simulink library "halin"  (R2021b)
settings: Solver=VariableStepAuto  StartTime=0.0  StopTime=10.0  RelTol=1e-3
undefined symbols (not defined in the file): KHAL_CAN1ABM1E2E_flg, KHAL_CAN1EPB1E2E_flg, KHAL_CAN1EPS1E2E_flg, KHAL_CAN1ESC1E2E_flg, KHAL_CAN1ESC5E2E_flg, KHAL_CAN3BMS1E2E_flg, KHAL_CAN3BMS6E2E_flg, KHAL_CAN3CCU1E2E_flg, KHAL_CAN3CCU2E2E_flg, KHAL_CAN3MCUNF1E2E_flg, KHAL_CAN3MCUNR1E2E_flg, KHAL_CAN3Shifter1E2E_flg, KHAL_CAN3Shifter2E2E_flg, KHAL_CAN6FCM2E2E_flg, KHAL_CAN6FCM4E2E_flg, TRUE
libraries: simulink x645, FVT_lib x212, hcu_lib x59
(part 23 of 23)

== system halin/HAL_IN/CAN6/FCM1/ForceLowBeam ==
  ForceLowBeam : Inport
  UnitConverter : DataTypeConversion  OutDataTypeStr=uint8
  VHAL_ForceLowBeam_enum : Outport
  wires:
  UnitConverter/1 -> VHAL_ForceLowBeam_enum/1
  ForceLowBeam/1 -> UnitConverter/1

== system halin/HAL_IN/CAN6/FCM1/HazardWarningReq ==
  HazardWarningReq : Inport
  UnitConverter : DataTypeConversion  OutDataTypeStr=uint8
  VHAL_HazardWarningReq_flg : Outport
  wires:
  UnitConverter/1 -> VHAL_HazardWarningReq_flg/1
  HazardWarningReq/1 -> UnitConverter/1

== system halin/HAL_IN/CAN6/FCM1/ISAWarningMsg ==
  ISA_WarningMsg : Inport
  UnitConverter : DataTypeConversion  OutDataTypeStr=uint8
  VHAL_ISAWarningMsg_enum : Outport
  wires:
  UnitConverter/1 -> VHAL_ISAWarningMsg_enum/1
  ISA_WarningMsg/1 -> UnitConverter/1

== system halin/HAL_IN/CAN6/FCM1/LKAHODDisplayWarning ==
  LKA_HOD_Display_Warning : Inport
  UnitConverter : DataTypeConversion  OutDataTypeStr=uint8
  VHAL_LKAHODDisplayWarning_flg : Outport
  wires:
  UnitConverter/1 -> VHAL_LKAHODDisplayWarning_flg/1
  LKA_HOD_Display_Warning/1 -> UnitConverter/1

== system halin/HAL_IN/CAN6/FCM1/LKAHODSoundWarning ==
  LKA_HOD_Sound_Warning : Inport
  UnitConverter : DataTypeConversion  OutDataTypeStr=uint8
  VHAL_LKAHODSoundWarning_flg : Outport
  wires:
  UnitConverter/1 -> VHAL_LKAHODSoundWarning_flg/1
  LKA_HOD_Sound_Warning/1 -> UnitConverter/1

== system halin/HAL_IN/CAN6/FCM1/LVDAACCStatusInformation ==
  LVDA_ACCStatusInformation : Inport
  UnitConverter : DataTypeConversion  OutDataTypeStr=uint8
  VHAL_LVDAACCStatusInformation_flg : Outport
  wires:
  UnitConverter/1 -> VHAL_LVDAACCStatusInformation_flg/1
  LVDA_ACCStatusInformation/1 -> UnitConverter/1

== system halin/HAL_IN/CAN6/FCM1/LVDADisabled ==
  LVDA_Disabled : Inport
  UnitConverter : DataTypeConversion  OutDataTypeStr=uint8
  VHAL_LVDADisabled_flg : Outport
  wires:
  UnitConverter/1 -> VHAL_LVDADisabled_flg/1
  LVDA_Disabled/1 -> UnitConverter/1

== system halin/HAL_IN/CAN6/FCM1/LVDAFailinfo ==
  LVDA_Failinfo : Inport
  UnitConverter : DataTypeConversion  OutDataTypeStr=uint8
  VHAL_LVDAFailinfo_flg : Outport
  wires:
  UnitConverter/1 -> VHAL_LVDAFailinfo_flg/1
  LVDA_Failinfo/1 -> UnitConverter/1

== system halin/HAL_IN/CAN6/FCM1/LVDAMuteSta ==
  LVDA_Mute_Sta : Inport
  UnitConverter : DataTypeConversion  OutDataTypeStr=uint8
  VHAL_LVDAMuteSta_enum : Outport
  wires:
  UnitConverter/1 -> VHAL_LVDAMuteSta_enum/1
  LVDA_Mute_Sta/1 -> UnitConverter/1

== system halin/HAL_IN/CAN6/FCM1/LVDAWarning ==
  LVDA_Warning : Inport
  UnitConverter : DataTypeConversion  OutDataTypeStr=uint8
  VHAL_LVDAWarning_flg : Outport
  wires:
  UnitConverter/1 -> VHAL_LVDAWarning_flg/1
  LVDA_Warning/1 -> UnitConverter/1

== system halin/HAL_IN/CAN6/FCM1/LeftTurnLightReq ==
  LeftTurnLightReq : Inport
  UnitConverter : DataTypeConversion  OutDataTypeStr=uint8
  VHAL_LeftTurnLightReq_flg : Outport
  wires:
  UnitConverter/1 -> VHAL_LeftTurnLightReq_flg/1
  LeftTurnLightReq/1 -> UnitConverter/1

== system halin/HAL_IN/CAN6/FCM1/RightTurnLightReq ==
  RightTurnLightReq : Inport
  UnitConverter : DataTypeConversion  OutDataTypeStr=uint8
  VHAL_RightTurnLightReq_flg : Outport
  wires:
  UnitConverter/1 -> VHAL_RightTurnLightReq_flg/1
  RightTurnLightReq/1 -> UnitConverter/1

== system halin/HAL_IN/CAN6/FCM1/TargetType ==
  Target_Type : Inport
  UnitConverter : DataTypeConversion  OutDataTypeStr=uint16
  VHAL_TargetType_enum : Outport
  wires:
  UnitConverter/1 -> VHAL_TargetType_enum/1
  Target_Type/1 -> UnitConverter/1

== system halin/HAL_IN/CAN6/FCM1/TimeGapLevel ==
  TimeGapLevel : Inport
  UnitConverter : DataTypeConversion  OutDataTypeStr=uint8
  VHAL_TimeGapLevel_enum : Outport
  wires:
  UnitConverter/1 -> VHAL_TimeGapLevel_enum/1
  TimeGapLevel/1 -> UnitConverter/1

== system halin/HAL_IN/CAN6/FCM2/ADBVehDst1Val ==
  ADB_VehDst1Val : Inport
  UnitConverter : DataTypeConversion  OutDataTypeStr=uint8
  VHAL_ADBVehDst1Val_enum : Outport
  wires:
  UnitConverter/1 -> VHAL_ADBVehDst1Val_enum/1
  ADB_VehDst1Val/1 -> UnitConverter/1

== system halin/HAL_IN/CAN6/FCM3/MELaneCurvDervLt ==
  ME_Lane_CurvDervLt : Inport
  UnitConverter : DataTypeConversion  OutDataTypeStr=uint16
  convert_in : FVT_lib/hal/convert_in  gain=4e-09  offset=-0.00013
  VHAL_MELaneCurvDervLt_raw32 : Outport
  wires:
  convert_in/1 -> VHAL_MELaneCurvDervLt_raw32/1
  UnitConverter/1 -> convert_in/1
  ME_Lane_CurvDervLt/1 -> UnitConverter/1

== system halin/HAL_IN/CAN6/FCM3/MELaneCurvDervLt2 ==
  ME_Lane_CurvDervLt2 : Inport
  UnitConverter : DataTypeConversion  OutDataTypeStr=uint16
  convert_in : FVT_lib/hal/convert_in  gain=4e-09  offset=-0.00013
  VHAL_MELaneCurvDervLt2_raw32 : Outport
  wires:
  convert_in/1 -> VHAL_MELaneCurvDervLt2_raw32/1
  UnitConverter/1 -> convert_in/1
  ME_Lane_CurvDervLt2/1 -> UnitConverter/1

== system halin/HAL_IN/CAN6/FCM3/MELaneCurvDervRt ==
  ME_Lane_CurvDervRt : Inport
  UnitConverter : DataTypeConversion  OutDataTypeStr=uint16
  convert_in : FVT_lib/hal/convert_in  gain=4e-09  offset=-0.00013
  VHAL_MELaneCurvDervRt_raw32 : Outport
  wires:
  convert_in/1 -> VHAL_MELaneCurvDervRt_raw32/1
  UnitConverter/1 -> convert_in/1
  ME_Lane_CurvDervRt/1 -> UnitConverter/1

== system halin/HAL_IN/CAN6/FCM3/MELaneCurvDervRt2 ==
  ME_Lane_CurvDervRt2 : Inport
  UnitConverter : DataTypeConversion  OutDataTypeStr=uint16
  convert_in : FVT_lib/hal/convert_in  gain=4e-09  offset=-0.00013
  VHAL_MELaneCurvDervRt2_raw32 : Outport
  wires:
  convert_in/1 -> VHAL_MELaneCurvDervRt2_raw32/1
  UnitConverter/1 -> convert_in/1
  ME_Lane_CurvDervRt2/1 -> UnitConverter/1

== system halin/HAL_IN/CAN6/FCM3/MELaneCurvLt ==
  ME_Lane_CurvLt : Inport
  UnitConverter : DataTypeConversion  OutDataTypeStr=uint16
  convert_in : FVT_lib/hal/convert_in  gain=1e-06  offset=-0.032
  VHAL_MELaneCurvLt_raw32 : Outport
  wires:
  convert_in/1 -> VHAL_MELaneCurvLt_raw32/1
  UnitConverter/1 -> convert_in/1
  ME_Lane_CurvLt/1 -> UnitConverter/1

== system halin/HAL_IN/CAN6/FCM3/MELaneCurvLt2 ==
  ME_Lane_CurvLt2 : Inport
  UnitConverter : DataTypeConversion  OutDataTypeStr=uint16
  convert_in : FVT_lib/hal/convert_in  gain=1e-06  offset=-0.032
  VHAL_MELaneCurvLt2_raw32 : Outport
  wires:
  convert_in/1 -> VHAL_MELaneCurvLt2_raw32/1
  UnitConverter/1 -> convert_in/1
  ME_Lane_CurvLt2/1 -> UnitConverter/1

== system halin/HAL_IN/CAN6/FCM3/MELaneCurvRt ==
  ME_Lane_CurvRt : Inport
  UnitConverter : DataTypeConversion  OutDataTypeStr=uint16
  convert_in : FVT_lib/hal/convert_in  gain=1e-06  offset=-0.032
  VHAL_MELaneCurvRt_raw32 : Outport
  wires:
  convert_in/1 -> VHAL_MELaneCurvRt_raw32/1
  UnitConverter/1 -> convert_in/1
  ME_Lane_CurvRt/1 -> UnitConverter/1

== system halin/HAL_IN/CAN6/FCM3/MELaneCurvRt2 ==
  ME_Lane_CurvRt2 : Inport
  UnitConverter : DataTypeConversion  OutDataTypeStr=uint16
  convert_in : FVT_lib/hal/convert_in  gain=1e-06  offset=-0.032
  VHAL_MELaneCurvRt2_raw32 : Outport
  wires:
  convert_in/1 -> VHAL_MELaneCurvRt2_raw32/1
  UnitConverter/1 -> convert_in/1
  ME_Lane_CurvRt2/1 -> UnitConverter/1

== system halin/HAL_IN/CAN6/FCM3/MELaneHeadAngLt ==
  ME_Lane_HeadAngLt : Inport
  UnitConverter : DataTypeConversion  OutDataTypeStr=uint16
  convert_in : FVT_lib/hal/convert_in  gain=0.001  offset=-0.5
  VHAL_MELaneHeadAngLt_radians : Outport
  wires:
  convert_in/1 -> VHAL_MELaneHeadAngLt_radians/1
  UnitConverter/1 -> convert_in/1
  ME_Lane_HeadAngLt/1 -> UnitConverter/1

== system halin/HAL_IN/CAN6/FCM3/MELaneHeadAngLt2 ==
  ME_Lane_HeadAngLt2 : Inport
  UnitConverter : DataTypeConversion  OutDataTypeStr=uint16
  convert_in : FVT_lib/hal/convert_in  gain=0.001  offset=-0.5
  VHAL_MELaneHeadAngLt2_radians : Outport
  wires:
  convert_in/1 -> VHAL_MELaneHeadAngLt2_radians/1
  UnitConverter/1 -> convert_in/1
  ME_Lane_HeadAngLt2/1 -> UnitConverter/1

== system halin/HAL_IN/CAN6/FCM3/MELaneHeadAngRt ==
  ME_Lane_HeadAngRt : Inport
  UnitConverter : DataTypeConversion  OutDataTypeStr=uint16
  convert_in : FVT_lib/hal/convert_in  gain=0.001  offset=-0.5
  VHAL_MELaneHeadAngRt_radians : Outport
  wires:
  convert_in/1 -> VHAL_MELaneHeadAngRt_radians/1
  UnitConverter/1 -> convert_in/1
  ME_Lane_HeadAngRt/1 -> UnitConverter/1

== system halin/HAL_IN/CAN6/FCM3/MELaneHeadAngRt2 ==
  ME_Lane_HeadAngRt2 : Inport
  UnitConverter : DataTypeConversion  OutDataTypeStr=uint16
  convert_in : FVT_lib/hal/convert_in  gain=0.001  offset=-0.5
  VHAL_MELaneHeadAngRt2_radians : Outport
  wires:
  convert_in/1 -> VHAL_MELaneHeadAngRt2_radians/1
  UnitConverter/1 -> convert_in/1
  ME_Lane_HeadAngRt2/1 -> UnitConverter/1

== system halin/HAL_IN/CAN6/FCM3/MELanePosLt ==
  ME_Lane_PosLt : Inport
  UnitConverter : DataTypeConversion  OutDataTypeStr=uint16
  convert_in : FVT_lib/hal/convert_in  gain=0.01  offset=-10
  VHAL_MELanePosLt_m : Outport
  wires:
  convert_in/1 -> VHAL_MELanePosLt_m/1
  UnitConverter/1 -> convert_in/1
  ME_Lane_PosLt/1 -> UnitConverter/1

== system halin/HAL_IN/CAN6/FCM3/MELanePosLt2 ==
  ME_Lane_PosLt2 : Inport
  UnitConverter : DataTypeConversion  OutDataTypeStr=uint16
  convert_in : FVT_lib/hal/convert_in  gain=0.01  offset=-10
  VHAL_MELanePosLt2_m : Outport
  wires:
  convert_in/1 -> VHAL_MELanePosLt2_m/1
  UnitConverter/1 -> convert_in/1
  ME_Lane_PosLt2/1 -> UnitConverter/1

== system halin/HAL_IN/CAN6/FCM3/MELanePosRt ==
  ME_Lane_PosRt : Inport
  UnitConverter : DataTypeConversion  OutDataTypeStr=uint16
  convert_in : FVT_lib/hal/convert_in  gain=0.01  offset=-10
  VHAL_MELanePosRt_m : Outport
  wires:
  convert_in/1 -> VHAL_MELanePosRt_m/1
  UnitConverter/1 -> convert_in/1
  ME_Lane_PosRt/1 -> UnitConverter/1

== system halin/HAL_IN/CAN6/FCM3/MELanePosRt2 ==
  ME_Lane_PosRt2 : Inport
  UnitConverter : DataTypeConversion  OutDataTypeStr=uint16
  convert_in : FVT_lib/hal/convert_in  gain=0.01  offset=-10
  VHAL_MELanePosRt2_m : Outport
  wires:
  convert_in/1 -> VHAL_MELanePosRt2_m/1
  UnitConverter/1 -> convert_in/1
  ME_Lane_PosRt2/1 -> UnitConverter/1

== system halin/HAL_IN/CAN6/FCM4/ADASAngCtrlTqWeightGain ==
  ADAS_AngCtrlTqWeightGain : Inport
  UnitConverter : DataTypeConversion  OutDataTypeStr=uint8
  convert_in : FVT_lib/hal/convert_in  gain=0.4  offset=0
  VHAL_ADASAngCtrlTqWeightGain_pct : Outport
  wires:
  convert_in/1 -> VHAL_ADASAngCtrlTqWeightGain_pct/1
  UnitConverter/1 -> convert_in/1
  ADAS_AngCtrlTqWeightGain/1 -> UnitConverter/1

== system halin/HAL_IN/CAN6/FCM4/ADASDesStrWhlAngCtrlCmd ==
  ADAS_DesStrWhlAngCtrlCmd : Inport
  UnitConverter : DataTypeConversion  OutDataTypeStr=uint16
  convert_in : FVT_lib/hal/convert_in  gain=0.1  offset=-900
  VHAL_ADASDesStrWhlAngCtrlCmd_Deg : Outport
  wires:
  convert_in/1 -> VHAL_ADASDesStrWhlAngCtrlCmd_Deg/1
  UnitConverter/1 -> convert_in/1
  ADAS_DesStrWhlAngCtrlCmd/1 -> UnitConverter/1

== system halin/HAL_IN/CAN6/FCM4/ADASDrvInputTqBoostAct ==
  ADAS_DrvInputTqBoostAct : Inport
  UnitConverter : DataTypeConversion  OutDataTypeStr=uint8
  VHAL_ADASDrvInputTqBoostAct_flg : Outport
  wires:
  UnitConverter/1 -> VHAL_ADASDrvInputTqBoostAct_flg/1
  ADAS_DrvInputTqBoostAct/1 -> UnitConverter/1

== system halin/HAL_IN/CAN6/FCM4/ADASDrvInputTqBoostGain ==
  ADAS_DrvInputTqBoostGain : Inport
  UnitConverter : DataTypeConversion  OutDataTypeStr=uint8
  convert_in : FVT_lib/hal/convert_in  gain=0.4  offset=0
  VHAL_ADASDrvInputTqBoostGain_pct : Outport
  wires:
  convert_in/1 -> VHAL_ADASDrvInputTqBoostGain_pct/1
  UnitConverter/1 -> convert_in/1
  ADAS_DrvInputTqBoostGain/1 -> UnitConverter/1

== system halin/HAL_IN/CAN6/FCM4/ADASMaxAngCtrlOutTqLimit ==
  ADAS_MaxAngCtrlOutTqLimit : Inport
  UnitConverter : DataTypeConversion  OutDataTypeStr=uint16
  convert_in : FVT_lib/hal/convert_in  gain=0.1  offset=0
  VHAL_ADASMaxAngCtrlOutTqLimit_Nm : Outport
  wires:
  convert_in/1 -> VHAL_ADASMaxAngCtrlOutTqLimit_Nm/1
  UnitConverter/1 -> convert_in/1
  ADAS_MaxAngCtrlOutTqLimit/1 -> UnitConverter/1

== system halin/HAL_IN/CAN6/FCM4/ADASStrWhlAngCtrlStatus ==
  ADAS_StrWhlAngCtrlStatus : Inport
  UnitConverter : DataTypeConversion  OutDataTypeStr=uint8
  VHAL_ADASStrWhlAngCtrlStatus_flg : Outport
  wires:
  UnitConverter/1 -> VHAL_ADASStrWhlAngCtrlStatus_flg/1
  ADAS_StrWhlAngCtrlStatus/1 -> UnitConverter/1

== system halin/HAL_IN/CAN6/SRR1/SRRBSDWarnL ==
  SRR_BSD_WarnL : Inport
  UnitConverter : DataTypeConversion  OutDataTypeStr=uint8
  VHAL_SRRBSDWarnL_enum : Outport
  wires:
  UnitConverter/1 -> VHAL_SRRBSDWarnL_enum/1
  SRR_BSD_WarnL/1 -> UnitConverter/1

== system halin/HAL_IN/CAN6/SRR1/SRRBSDWarnR ==
  SRR_BSD_WarnR : Inport
  UnitConverter : DataTypeConversion  OutDataTypeStr=uint8
  VHAL_SRRBSDWarnR_enum : Outport
  wires:
  UnitConverter/1 -> VHAL_SRRBSDWarnR_enum/1
  SRR_BSD_WarnR/1 -> UnitConverter/1

== system halin/HAL_IN/CAN6/SRR1/SRRODASoundL ==
  SRR_ODA_SoundL : Inport
  UnitConverter : DataTypeConversion  OutDataTypeStr=uint8
  VHAL_SRRODASoundL_flg : Outport
  wires:
  UnitConverter/1 -> VHAL_SRRODASoundL_flg/1
  SRR_ODA_SoundL/1 -> UnitConverter/1

== system halin/HAL_IN/CAN6/SRR1/SRRODASoundR ==
  SRR_ODA_SoundR : Inport
  UnitConverter : DataTypeConversion  OutDataTypeStr=uint8
  VHAL_SRRODASoundR_flg : Outport
  wires:
  UnitConverter/1 -> VHAL_SRRODASoundR_flg/1
  SRR_ODA_SoundR/1 -> UnitConverter/1

== system halin/HAL_IN/CAN6/SRR1/SRRODAWarnL ==
  SRR_ODA_WarnL : Inport
  UnitConverter : DataTypeConversion  OutDataTypeStr=uint8
  VHAL_SRRODAWarnL_enum : Outport
  wires:
  UnitConverter/1 -> VHAL_SRRODAWarnL_enum/1
  SRR_ODA_WarnL/1 -> UnitConverter/1

== system halin/HAL_IN/CAN6/SRR1/SRRODAWarnR ==
  SRR_ODA_WarnR : Inport
  UnitConverter : DataTypeConversion  OutDataTypeStr=uint8
  VHAL_SRRODAWarnR_enum : Outport
  wires:
  UnitConverter/1 -> VHAL_SRRODAWarnR_enum/1
  SRR_ODA_WarnR/1 -> UnitConverter/1
